simulink model "c2837xD_lcd_display"  (R2021b)
settings: Solver=FixedStepDiscrete  StartTime=0.0  StopTime=Inf  RelTol=1e-3  EnableMultiTasking=on
InitFcn:
  | c2837xD_Display_Param;
values from neighbouring files (symbols this model uses):
  SCI_counter = SCI_ping_buffer_size/SCI_chunk_size    (= 640)    [c2837xD_Display_Param.m]
  SCI_ping_buffer_size = image_height*lines_in_packet    (= 3840)    [c2837xD_Display_Param.m]
  TI_chunk_size = SCI_chunk_size    (= 6)    [c2837xD_Display_Param.m]
  TI_ping_buffer_size = SCI_ping_buffer_size    (= 3840)    [c2837xD_Display_Param.m]
libraries: c280xlib x63, c2837xDlib x63, simulink x41, c2000lib x1, demo_controls x1, dspswit3 x1, idelinklib_common x1
(part 4 of 4)

== system c2837xD_lcd_display/Initialization/VCOM_OTP_1_REG/Subsystem/SetData ==
  function : TriggerPort  TriggerType=function-call  VariantControl=Variant
  Constant1 : Constant  SampleTime=-1
  Digital Output1 : c2837xDlib/Digital Output  GPIO_Number=GPIO16~GPIO23  GPIO_Bit0=off  GPIO_BIT0_Toggle=off  GPIO_Bit1=off  GPIO_BIT1_Toggle=off  GPIO_Bit2=off  GPIO_BIT2_Toggle=off  GPIO_Bit3=off  GPIO_BIT3_Toggle=off  GPIO_Bit4=off  GPIO_BIT4_Toggle=off  GPIO_Bit5=off  GPIO_BIT5_Toggle=off  GPIO_Bit6=on  GPIO_BIT6_Toggle=off  GPIO_Bit7=off  GPIO_BIT7_Toggle=off
      settings: SourceProductBaseCode=TIC2000
  wires:
  Constant1/1 -> Digital Output1/1

== system c2837xD_lcd_display/Initialization/Volt6p1/Subsystem/SendCommand ==
  cmd : Inport
  function : TriggerPort  TriggerType=function-call  VariantControl=Variant
  SPI Master Transfer : c280xlib/SPI Master Transfer  SPISelect=SPI_A  ClockPolarity=Rising_edge  ClockPhase=Delay_half_cycle  SPIModule=uint32(0)  Mode=Master  BusSpeed=uint32(1000000)  FirstBitToTransfer=Most significant bit (MSB)  ClockMode=0  BlockFunction=Transfer  EnableRegisterAddress=off  RegisterAddress=0  OutputDataType=int8  OutputDataLength=1  DataBits=8  UseCustomSSPin=Explicit GPIO calls  ActiveLowSSPin=Active low  Pin=124
      settings: SourceProductBaseCode=TIC2000
  Terminator : Terminator
  wires:
  cmd/1 -> SPI Master Transfer/1
  SPI Master Transfer/1 -> Terminator/1

== system c2837xD_lcd_display/Initialization/Volt6p1/Subsystem/SendData ==
  Data : Inport
  function : TriggerPort  TriggerType=function-call  VariantControl=Variant
  SPI Master Transfer : c280xlib/SPI Master Transfer  SPISelect=SPI_A  ClockPolarity=Rising_edge  ClockPhase=Delay_half_cycle  SPIModule=uint32(0)  Mode=Master  BusSpeed=uint32(1000000)  FirstBitToTransfer=Most significant bit (MSB)  ClockMode=0  BlockFunction=Transfer  EnableRegisterAddress=off  RegisterAddress=0  OutputDataType=int8  OutputDataLength=1  DataBits=8  UseCustomSSPin=Explicit GPIO calls  ActiveLowSSPin=Active low  Pin=124
      settings: SourceProductBaseCode=TIC2000
  Terminator : Terminator
  wires:
  Data/1 -> SPI Master Transfer/1
  SPI Master Transfer/1 -> Terminator/1

== system c2837xD_lcd_display/Initialization/Volt6p1/Subsystem/SetCmd ==
  function : TriggerPort  TriggerType=function-call  VariantControl=Variant
  Constant : Constant  Value=0  SampleTime=-1
  Digital Output : c2837xDlib/Digital Output  GPIO_Number=GPIO16~GPIO23  GPIO_Bit0=off  GPIO_BIT0_Toggle=off  GPIO_Bit1=off  GPIO_BIT1_Toggle=off  GPIO_Bit2=off  GPIO_BIT2_Toggle=off  GPIO_Bit3=off  GPIO_BIT3_Toggle=off  GPIO_Bit4=off  GPIO_BIT4_Toggle=off  GPIO_Bit5=off  GPIO_BIT5_Toggle=off  GPIO_Bit6=on  GPIO_BIT6_Toggle=off  GPIO_Bit7=off  GPIO_BIT7_Toggle=off
      settings: SourceProductBaseCode=TIC2000
  wires:
  Constant/1 -> Digital Output/1

== system c2837xD_lcd_display/Initialization/Volt6p1/Subsystem/SetData ==
  function : TriggerPort  TriggerType=function-call  VariantControl=Variant
  Constant1 : Constant  SampleTime=-1
  Digital Output1 : c2837xDlib/Digital Output  GPIO_Number=GPIO16~GPIO23  GPIO_Bit0=off  GPIO_BIT0_Toggle=off  GPIO_Bit1=off  GPIO_BIT1_Toggle=off  GPIO_Bit2=off  GPIO_BIT2_Toggle=off  GPIO_Bit3=off  GPIO_BIT3_Toggle=off  GPIO_Bit4=off  GPIO_BIT4_Toggle=off  GPIO_Bit5=off  GPIO_BIT5_Toggle=off  GPIO_Bit6=on  GPIO_BIT6_Toggle=off  GPIO_Bit7=off  GPIO_BIT7_Toggle=off
      settings: SourceProductBaseCode=TIC2000
  wires:
  Constant1/1 -> Digital Output1/1

== system c2837xD_lcd_display/Initialization/Volt6p2/Subsystem/SendCommand ==
  cmd : Inport
  function : TriggerPort  TriggerType=function-call  VariantControl=Variant
  SPI Master Transfer : c280xlib/SPI Master Transfer  SPISelect=SPI_A  ClockPolarity=Rising_edge  ClockPhase=Delay_half_cycle  SPIModule=uint32(0)  Mode=Master  BusSpeed=uint32(1000000)  FirstBitToTransfer=Most significant bit (MSB)  ClockMode=0  BlockFunction=Transfer  EnableRegisterAddress=off  RegisterAddress=0  OutputDataType=int8  OutputDataLength=1  DataBits=8  UseCustomSSPin=Explicit GPIO calls  ActiveLowSSPin=Active low  Pin=124
      settings: SourceProductBaseCode=TIC2000
  Terminator : Terminator
  wires:
  cmd/1 -> SPI Master Transfer/1
  SPI Master Transfer/1 -> Terminator/1

== system c2837xD_lcd_display/Initialization/Volt6p2/Subsystem/SendData ==
  Data : Inport
  function : TriggerPort  TriggerType=function-call  VariantControl=Variant
  SPI Master Transfer : c280xlib/SPI Master Transfer  SPISelect=SPI_A  ClockPolarity=Rising_edge  ClockPhase=Delay_half_cycle  SPIModule=uint32(0)  Mode=Master  BusSpeed=uint32(1000000)  FirstBitToTransfer=Most significant bit (MSB)  ClockMode=0  BlockFunction=Transfer  EnableRegisterAddress=off  RegisterAddress=0  OutputDataType=int8  OutputDataLength=1  DataBits=8  UseCustomSSPin=Explicit GPIO calls  ActiveLowSSPin=Active low  Pin=124
      settings: SourceProductBaseCode=TIC2000
  Terminator : Terminator
  wires:
  Data/1 -> SPI Master Transfer/1
  SPI Master Transfer/1 -> Terminator/1

== system c2837xD_lcd_display/Initialization/Volt6p2/Subsystem/SetCmd ==
  function : TriggerPort  TriggerType=function-call  VariantControl=Variant
  Constant : Constant  Value=0  SampleTime=-1
  Digital Output : c2837xDlib/Digital Output  GPIO_Number=GPIO16~GPIO23  GPIO_Bit0=off  GPIO_BIT0_Toggle=off  GPIO_Bit1=off  GPIO_BIT1_Toggle=off  GPIO_Bit2=off  GPIO_BIT2_Toggle=off  GPIO_Bit3=off  GPIO_BIT3_Toggle=off  GPIO_Bit4=off  GPIO_BIT4_Toggle=off  GPIO_Bit5=off  GPIO_BIT5_Toggle=off  GPIO_Bit6=on  GPIO_BIT6_Toggle=off  GPIO_Bit7=off  GPIO_BIT7_Toggle=off
      settings: SourceProductBaseCode=TIC2000
  wires:
  Constant/1 -> Digital Output/1

== system c2837xD_lcd_display/Initialization/Volt6p2/Subsystem/SetData ==
  function : TriggerPort  TriggerType=function-call  VariantControl=Variant
  Constant1 : Constant  SampleTime=-1
  Digital Output1 : c2837xDlib/Digital Output  GPIO_Number=GPIO16~GPIO23  GPIO_Bit0=off  GPIO_BIT0_Toggle=off  GPIO_Bit1=off  GPIO_BIT1_Toggle=off  GPIO_Bit2=off  GPIO_BIT2_Toggle=off  GPIO_Bit3=off  GPIO_BIT3_Toggle=off  GPIO_Bit4=off  GPIO_BIT4_Toggle=off  GPIO_Bit5=off  GPIO_BIT5_Toggle=off  GPIO_Bit6=on  GPIO_BIT6_Toggle=off  GPIO_Bit7=off  GPIO_BIT7_Toggle=off
      settings: SourceProductBaseCode=TIC2000
  wires:
  Constant1/1 -> Digital Output1/1

== system c2837xD_lcd_display/Initialization/Volt6p2/Subsystem1/SendCommand ==
  cmd : Inport
  function : TriggerPort  TriggerType=function-call  VariantControl=Variant
  SPI Master Transfer : c280xlib/SPI Master Transfer  SPISelect=SPI_A  ClockPolarity=Rising_edge  ClockPhase=Delay_half_cycle  SPIModule=uint32(0)  Mode=Master  BusSpeed=uint32(1000000)  FirstBitToTransfer=Most significant bit (MSB)  ClockMode=0  BlockFunction=Transfer  EnableRegisterAddress=off  RegisterAddress=0  OutputDataType=int8  OutputDataLength=1  DataBits=8  UseCustomSSPin=Explicit GPIO calls  ActiveLowSSPin=Active low  Pin=124
      settings: SourceProductBaseCode=TIC2000
  Terminator : Terminator
  wires:
  cmd/1 -> SPI Master Transfer/1
  SPI Master Transfer/1 -> Terminator/1

== system c2837xD_lcd_display/Initialization/Volt6p2/Subsystem1/SendData ==
  Data : Inport
  function : TriggerPort  TriggerType=function-call  VariantControl=Variant
  SPI Master Transfer : c280xlib/SPI Master Transfer  SPISelect=SPI_A  ClockPolarity=Rising_edge  ClockPhase=Delay_half_cycle  SPIModule=uint32(0)  Mode=Master  BusSpeed=uint32(1000000)  FirstBitToTransfer=Most significant bit (MSB)  ClockMode=0  BlockFunction=Transfer  EnableRegisterAddress=off  RegisterAddress=0  OutputDataType=int8  OutputDataLength=1  DataBits=8  UseCustomSSPin=Explicit GPIO calls  ActiveLowSSPin=Active low  Pin=124
      settings: SourceProductBaseCode=TIC2000
  Terminator : Terminator
  wires:
  Data/1 -> SPI Master Transfer/1
  SPI Master Transfer/1 -> Terminator/1

== system c2837xD_lcd_display/Initialization/Volt6p2/Subsystem1/SetCmd ==
  function : TriggerPort  TriggerType=function-call  VariantControl=Variant
  Constant : Constant  Value=0  SampleTime=-1
  Digital Output : c2837xDlib/Digital Output  GPIO_Number=GPIO16~GPIO23  GPIO_Bit0=off  GPIO_BIT0_Toggle=off  GPIO_Bit1=off  GPIO_BIT1_Toggle=off  GPIO_Bit2=off  GPIO_BIT2_Toggle=off  GPIO_Bit3=off  GPIO_BIT3_Toggle=off  GPIO_Bit4=off  GPIO_BIT4_Toggle=off  GPIO_Bit5=off  GPIO_BIT5_Toggle=off  GPIO_Bit6=on  GPIO_BIT6_Toggle=off  GPIO_Bit7=off  GPIO_BIT7_Toggle=off
      settings: SourceProductBaseCode=TIC2000
  wires:
  Constant/1 -> Digital Output/1

== system c2837xD_lcd_display/Initialization/Volt6p2/Subsystem1/SetData ==
  function : TriggerPort  TriggerType=function-call  VariantControl=Variant
  Constant1 : Constant  SampleTime=-1
  Digital Output1 : c2837xDlib/Digital Output  GPIO_Number=GPIO16~GPIO23  GPIO_Bit0=off  GPIO_BIT0_Toggle=off  GPIO_Bit1=off  GPIO_BIT1_Toggle=off  GPIO_Bit2=off  GPIO_BIT2_Toggle=off  GPIO_Bit3=off  GPIO_BIT3_Toggle=off  GPIO_Bit4=off  GPIO_BIT4_Toggle=off  GPIO_Bit5=off  GPIO_BIT5_Toggle=off  GPIO_Bit6=on  GPIO_BIT6_Toggle=off  GPIO_Bit7=off  GPIO_BIT7_Toggle=off
      settings: SourceProductBaseCode=TIC2000
  wires:
  Constant1/1 -> Digital Output1/1

== system c2837xD_lcd_display/Serial_Interrupt/SCIInterruptEnable/ChangeStatus/ChangePongStatus ==
  IsPong : Inport
  function : TriggerPort  TriggerType=function-call  VariantControl=Variant
  Logical Operator : Logic  Operator=NOT  AllPortsSameDT=off  OutDataTypeStr=boolean
  SPI_PongStatus : Outport  InitialOutput=0  VectorParamsAs1DForOutWhenUnconnected=off
  wires:
  IsPong/1 -> Logical Operator/1
  Logical Operator/1 -> SPI_PongStatus/1

== system c2837xD_lcd_display/Serial_Interrupt/SCIInterruptEnable/ChangeStatus/EnableDMAInterrupt ==
  function : TriggerPort  TriggerType=function-call  VariantControl=Variant
  EnableDMAInterrupt : Subsystem  mask(System Outputs){ShowInLibBrowser=0}
      mask prompts: ShowInLibBrowser "Simulink:masks:CustCodeMaskParam1_MP"
      settings: CopyFcn=cccopyfcn(gcb)  OpenFcn=ccopenfcn('System Outputs Function')
      mask Help: eval('feval(''rtwprivate'',''rtwhelpview'',''rtw_sys_outputs_block'')');
      mask Display: disp('System\nOutputs');

== system c2837xD_lcd_display/Serial_Interrupt/SCIInterruptEnable/Counter Logic/SCI Counter ==
  DelimiterFoundStartCounting : Inport
  Compare To Constant : simulink/Logic and Bit Operations/Compare To Constant  relop=<  const=SCI_counter  OutDataTypeStr=boolean
  Counter : dspswit3/Counter  Direction=Up  CountEvent=Non-zero sample  CounterSize=16 bits  MaxCount=255  InitialCount=0  Output=Count  HitValue=32  ResetInput=on  SamplesPerFrame=1  Ts=-1  CntDtype=uint16  HitDtype=Logical
  Logical Operator2 : Logic  Operator=NOT  AllPortsSameDT=off  OutDataTypeStr=boolean
  Logical Operator6 : Logic  Operator=NOT  AllPortsSameDT=off  OutDataTypeStr=boolean
  Unit Delay2 : UnitDelay  InitialCondition=1  SampleTime=-1  HasFrameUpgradeWarning=on
  Counter_Value : Outport  VectorParamsAs1DForOutWhenUnconnected=off
  CounterReachedMax : Outport  Port=2  VectorParamsAs1DForOutWhenUnconnected=off
  wires:
  Compare To Constant/1 -> Logical Operator6/1, Unit Delay2/1  "Counter Still Counting"
  Unit Delay2/1 -> Logical Operator2/1
  Counter/1 -> Counter_Value/1, Compare To Constant/1
  Logical Operator6/1 -> CounterReachedMax/1
  Logical Operator2/1 -> Counter/2
  DelimiterFoundStartCounting/1 -> Counter/1

== system c2837xD_lcd_display/Serial_Interrupt/SCIInterruptEnable/Counter Logic/Search for Delimiter ==
  DelimiterMatching : Inport
  CounterReachedMax : Inport  Port=2
  Logical Operator2 : Logic  Operator=OR  AllPortsSameDT=off  OutDataTypeStr=boolean
  Logical Operator4 : Logic  AllPortsSameDT=off  OutDataTypeStr=boolean
  Logical Operator6 : Logic  Operator=NOT  AllPortsSameDT=off  OutDataTypeStr=boolean
  Unit Delay2 : UnitDelay  SampleTime=-1  HasFrameUpgradeWarning=on
  Delimiter_Found : Outport  VectorParamsAs1DForOutWhenUnconnected=off
  wires:
  CounterReachedMax/1 -> Logical Operator6/1
  DelimiterMatching/1 -> Logical Operator2/1
  Unit Delay2/1 -> Delimiter_Found/1, Logical Operator2/2  "search for delimiter"
  Logical Operator2/1 -> Logical Operator4/1
  Logical Operator4/1 -> Unit Delay2/1
  Logical Operator6/1 -> Logical Operator4/2

== system c2837xD_lcd_display/Serial_Interrupt/SCIInterruptEnable/Counter Logic/TogglePingPongStatus ==
  Enable : EnablePort
  Logical Operator1 : Logic  Operator=NOT  AllPortsSameDT=off  OutDataTypeStr=boolean
  Unit Delay : UnitDelay  InitialCondition=1  SampleTime=-1  HasFrameUpgradeWarning=on
  Out1 : Outport  InitialOutput=0  VectorParamsAs1DForOutWhenUnconnected=off
  wires:
  Unit Delay/1 -> Out1/1, Logical Operator1/1
  Logical Operator1/1 -> Unit Delay/1

== system c2837xD_lcd_display/Initialization/DataRegister/LCD Data/SendData/SendData ==
  Data1 : Inport
  For Iterator : ForIterator  IterationLimit=76800  ShowIterationPort=off  IndexMode=Zero-based
  SPI Master Transfer : c280xlib/SPI Master Transfer  SPISelect=SPI_A  ClockPolarity=Rising_edge  ClockPhase=Delay_half_cycle  SPIModule=uint32(0)  Mode=Master  BusSpeed=uint32(1000000)  FirstBitToTransfer=Most significant bit (MSB)  ClockMode=0  BlockFunction=Transfer  EnableRegisterAddress=off  RegisterAddress=0  OutputDataType=int8  OutputDataLength=1  DataBits=8  UseCustomSSPin=Explicit GPIO calls  ActiveLowSSPin=Active low  Pin=124
      settings: SourceProductBaseCode=TIC2000
  Terminator : Terminator
  wires:
  SPI Master Transfer/1 -> Terminator/1
  Data1/1 -> SPI Master Transfer/1

== system c2837xD_lcd_display/Serial_Interrupt/SCIInterruptEnable/ChangeStatus/EnableDMAInterrupt/EnableDMAInterrupt ==
